simulink model "Car_PRERL_Controller"  (R2023a)
settings: Solver=FixedStepAuto  StartTime=0.0  StopTime=40  FixedStep=0.01  RelTol=1e-3
values from neighbouring files (symbols this model uses):
  CS_PID_psi0 = 0    [Startup_CAR_SMC.m]
  CS_PID_psid0 = 0    [Startup_CAR_SMC.m]
  CS_PID_y0 = 0    [Startup_CAR_SMC.m]
  CS_PID_yd0 = 0    [Startup_CAR_SMC.m]
  Ctrl_Couple = (2*lf*Calpha_f)/Iz    (= 96.8054211036)    [Startup_CAR_SMC.m]
  PRERL_SMC_alpha = 0.01    [Startup_CAR_SMC.m]
  PRERL_SMC_beta = 0.15    [Startup_CAR_SMC.m]
  PRERL_SMC_delta_0 = 0.98    [Startup_CAR_SMC.m]
  PRERL_SMC_k = 1000000    [Startup_CAR_SMC.m]
  PRERL_SMC_lambda = 0.1    [Startup_CAR_SMC.m]
  PRERL_SMC_p = 0.01    [Startup_CAR_SMC.m]
undefined symbols (not defined in the file or in its folder): DiscIntNeverNeededParam
libraries: simulink x2
settings Model: Creator=Z0150218  LastModifiedBy=Z0150218

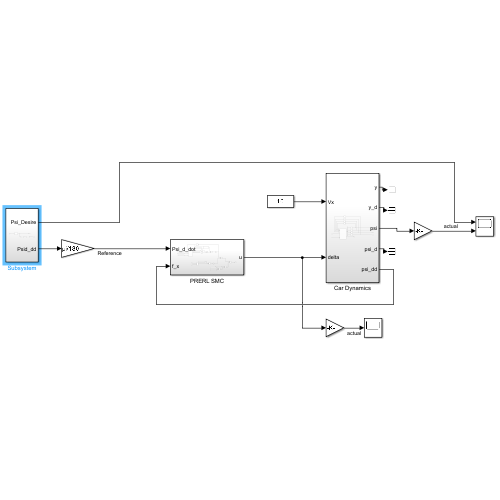
[thumbnail: Simulink's stored preview of the top-level diagram]
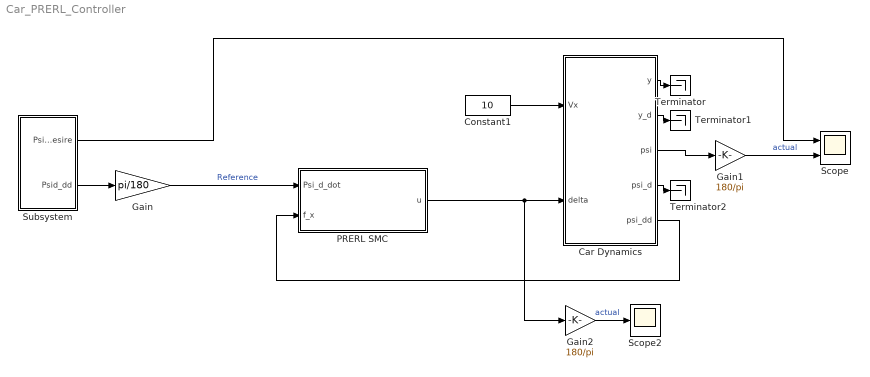
== system Car_PRERL_Controller ==
  Car Dynamics : Subsystem
  Constant1 : Constant  Value=10
  Gain : Gain  Gain=pi/180
  Gain1 : Gain  Gain=180/pi
  Gain2 : Gain  Gain=180/pi
  PRERL SMC : Subsystem
  Scope : Scope  NumInputPorts=2
  Scope2 : Scope
  Subsystem : Subsystem
  Terminator : Terminator
  Terminator1 : Terminator
  Terminator2 : Terminator
  wires:
  Gain2/1 -> Scope2/1  "actual"
  Gain1/1 -> Scope/2  "actual"
  Gain/1 -> PRERL SMC/1(Psi_d_dot)  "Reference"
  Subsystem/1(Psi_Desire) -> Scope/1
  Car Dynamics/4(psi_d) -> Terminator2/1
  Car Dynamics/3(psi) -> Gain1/1
  Car Dynamics/2(y_d) -> Terminator1/1
  Car Dynamics/1(y) -> Terminator/1
  Constant1/1 -> Car Dynamics/1(Vx)
  Subsystem/2(Psid_dd) -> Gain/1
  Car Dynamics/5(psi_dd) -> PRERL SMC/2(f_x)
  PRERL SMC/1(u) -> Gain2/1, Car Dynamics/2(delta)

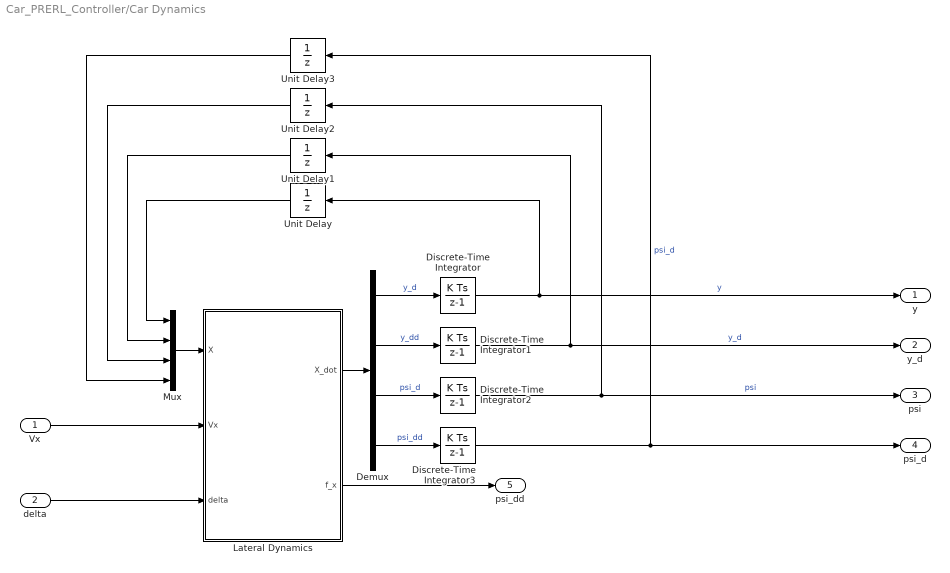
== system Car_PRERL_Controller/Car Dynamics ==
  Vx : Inport
  delta : Inport  Port=2
  Demux : Demux
  Discrete-Time Integrator{,1..3} (4 alike) : DiscreteIntegrator  SampleTime=-1  ICPrevOutput=DiscIntNeverNeededParam  ICPrevScaledInput=DiscIntNeverNeededParam
  Lateral Dynamics : MATLAB Function  TreatAsAtomicUnit=on
  Mux : Mux
  Unit Delay : UnitDelay  InitialCondition=CS_PID_y0  SampleTime=-1  HasFrameUpgradeWarning=on
  Unit Delay1 : UnitDelay  InitialCondition=CS_PID_yd0  SampleTime=-1  HasFrameUpgradeWarning=on
  Unit Delay2 : UnitDelay  InitialCondition=CS_PID_psi0  SampleTime=-1  HasFrameUpgradeWarning=on
  Unit Delay3 : UnitDelay  InitialCondition=CS_PID_psid0  SampleTime=-1  HasFrameUpgradeWarning=on
  y : Outport
  y_d : Outport  Port=2
  psi : Outport  Port=3
  psi_d : Outport  Port=4
  psi_dd : Outport  Port=5
  wires:
  Demux/1 -> Discrete-Time Integrator/1  "y_d"
  Unit Delay1/1 -> Mux/2
  Unit Delay3/1 -> Mux/4
  Discrete-Time Integrator/1 -> y/1, Unit Delay/1  "y"
  Mux/1 -> Lateral Dynamics/1(X)
  Lateral Dynamics/1(X_dot) -> Demux/1
  Discrete-Time Integrator3/1 -> psi_d/1, Unit Delay3/1  "psi_d"
  Discrete-Time Integrator1/1 -> y_d/1, Unit Delay1/1  "y_d"
  Vx/1 -> Lateral Dynamics/2(Vx)
  Unit Delay2/1 -> Mux/3
  Unit Delay/1 -> Mux/1
  Demux/3 -> Discrete-Time Integrator2/1  "psi_d"
  Demux/2 -> Discrete-Time Integrator1/1  "y_dd"
  Discrete-Time Integrator2/1 -> psi/1, Unit Delay2/1  "psi"
  Demux/4 -> Discrete-Time Integrator3/1  "psi_dd"
  delta/1 -> Lateral Dynamics/3(delta)
  Lateral Dynamics/2(f_x) -> psi_dd/1

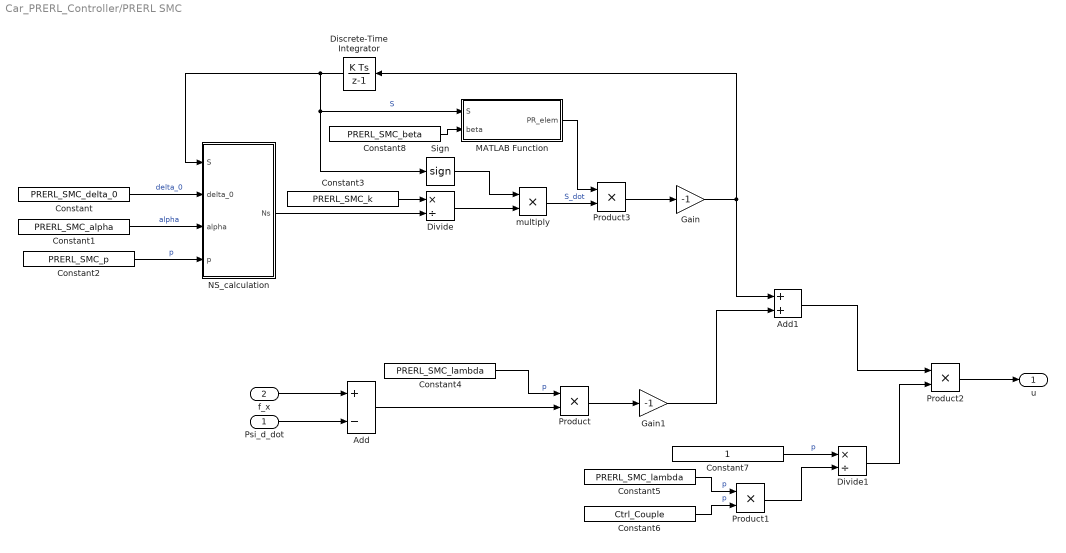
== system Car_PRERL_Controller/PRERL SMC ==
  Psi_d_dot : Inport
  f_x : Inport  Port=2
  Add : Sum  Inputs=+-
  Add1 : Sum
  Constant : Constant  Value=PRERL_SMC_delta_0
  Constant1 : Constant  Value=PRERL_SMC_alpha
  Constant2 : Constant  Value=PRERL_SMC_p
  Constant3 : Constant  Value=PRERL_SMC_k
  Constant4 : Constant  Value=PRERL_SMC_lambda
  Constant5 : Constant  Value=PRERL_SMC_lambda
  Constant6 : Constant  Value=Ctrl_Couple
  Constant7 : Constant
  Constant8 : Constant  Value=PRERL_SMC_beta
  Discrete-Time Integrator : DiscreteIntegrator  SampleTime=-1  ICPrevOutput=DiscIntNeverNeededParam  ICPrevScaledInput=DiscIntNeverNeededParam
  Divide : Product  Inputs=*/
  Divide1 : Product  Inputs=*/
  Gain : Gain  Gain=-1
  Gain1 : Gain  Gain=-1
  MATLAB Function : MATLAB Function  TreatAsAtomicUnit=on
  NS_calculation : MATLAB Function  TreatAsAtomicUnit=on
  Product{,1..3} (4 alike) : Product
  Sign : Signum
  multiply : Product  Inputs=**
  u : Outport
  wires:
  Discrete-Time Integrator/1 -> Sign/1, MATLAB Function/1(S), NS_calculation/1(S)  "S"
  multiply/1 -> Product3/2  "S_dot"
  f_x/1 -> Add/1
  Psi_d_dot/1 -> Add/2
  Constant/1 -> NS_calculation/2(delta_0)  "delta_0"
  Constant1/1 -> NS_calculation/3(alpha)  "alpha"
  Constant2/1 -> NS_calculation/4(p)  "p"
  Constant3/1 -> Divide/1
  NS_calculation/1(Ns) -> Divide/2
  Divide/1 -> multiply/2
  Sign/1 -> multiply/1
  Constant4/1 -> Product/1  "p"
  Add/1 -> Product/2
  Product/1 -> Gain1/1
  Gain/1 -> Add1/1, Discrete-Time Integrator/1
  Gain1/1 -> Add1/2
  Add1/1 -> Product2/1
  Constant5/1 -> Product1/1  "p"
  Constant6/1 -> Product1/2  "p"
  Constant7/1 -> Divide1/1  "p"
  Product1/1 -> Divide1/2
  Divide1/1 -> Product2/2
  Product2/1 -> u/1
  Constant8/1 -> MATLAB Function/2(beta)
  MATLAB Function/1(PR_elem) -> Product3/1
  Product3/1 -> Gain/1

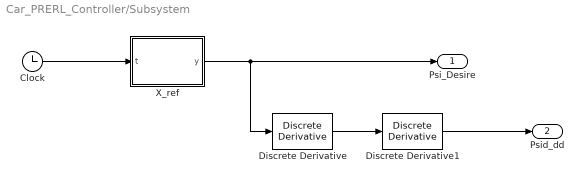
== system Car_PRERL_Controller/Subsystem ==
  Clock : Clock
  Discrete Derivative : simulink/Discrete/Discrete Derivative  gainval=1.0  ICPrevScaledInput=0.0  OutMin=[]  OutMax=[]  OutDataType=fixdt(1, 16)  OutScaling=2^-10  DoSatur=off
  Discrete Derivative1 : simulink/Discrete/Discrete Derivative  gainval=1.0  ICPrevScaledInput=0.0  OutMin=[]  OutMax=[]  OutDataType=fixdt(1, 16)  OutScaling=2^-10  DoSatur=off
  X_ref : MATLAB Function  TreatAsAtomicUnit=on
  Psi_Desire : Outport
  Psid_dd : Outport  Port=2
  wires:
  Clock/1 -> X_ref/1(t)
  X_ref/1(y) -> Discrete Derivative/1, Psi_Desire/1
  Discrete Derivative/1 -> Discrete Derivative1/1
  Discrete Derivative1/1 -> Psid_dd/1

== matlab function Car_PRERL_Controller/Subsystem/X_ref ==
  data: t input; y output
function y = fcn(t)
if t < 10
    y = 30;
elseif t >=10 && t <20
    y = -30;
else
    y = 30*sin(t);
end
end

== matlab function Car_PRERL_Controller/Car Dynamics/Lateral Dynamics ==
  data: X input; X_dot output; Vx input; delta input; f_x output
function [X_dot, f_x] = fcn(X,Vx,delta)

Calpha_f = 100000;
Calpha_r = 126000;
m = 2325;
Iz = 4132;
lr = 2;
lf = 2;

A22 = -((2*Calpha_f)+(2*Calpha_r))/(m*Vx);
A24 = -Vx - ((2*Calpha_f*lf)-(2*Calpha_r*lr))/(m*Vx);
A42 = -((2*lf*Calpha_f)-(2*lr*Calpha_r))/(Iz*Vx);
A44 = -((2*(lf^2)*Calpha_f)+(2*(lr^2)*Calpha_r))/(Iz*Vx);

B21 = 2*Calpha_f/m;
B41 = (2*lf*Calpha_f)/Iz;

A = [0 1 0 0; 0 A22 0 A24; 0 0 0 1; 0 A42 0 A44];
B = [0; B21; 0; B41];

X_dot = (A*X) + (B*delta);
f_xa   = (A*X);

f_x = f_xa(4);

== matlab function Car_PRERL_Controller/PRERL SMC/NS_calculation ==
  data: S input; Ns output; delta_0 input; alpha input; p input
function Ns = fcn(S, delta_0, alpha, p)

Ns = delta_0 + (1-delta_0)*exp(-alpha*abs(S)^p);
end

== matlab function Car_PRERL_Controller/PRERL SMC/MATLAB Function ==
  data: S input; PR_elem output; beta input
function PR_elem = fcn(S,beta)

PR_elem = abs(S)^beta;
end
